simulink model "altitude_controller"  (R2019b)
settings: Solver=ode45  StartTime=0.0  StopTime=50  FixedStep=1e-3  RelTol=1e-5
InitFcn:
  | % load parameters of the default quadrotor
  | disp('Quadrotor parameters loaded by InitFcn')
  | mdl_quadrotor
undefined symbols (not defined in the file or in its folder): A, B, C, D, pwm, quad
libraries: realtime_pacer_lib x2, simulink x1
settings Model: Creator=corkep  LastModifiedBy=lab
settings DataIOCC: LimitDataPoints=on  SaveFormat=Array  SignalLoggingSaveFormat=ModelDataLogs  ReturnWorkspaceOutputs=off
settings OptimizationCC: BlockReduction=off  BooleanDataType=off  LifeSpan=inf
settings DebuggingCC: SaveWithParameterizedLinksMsg=none  UnderspecifiedInitializationDetection=Classic  MergeDetectMultiDrivingBlocksExec=none  SignalResolutionControl=TryResolveAllWithWarning  MultiTaskDSMMsg=warning  MultiTaskCondExecSysMsg=none  AllowSymbolicDim=off  StateNameClashWarn=warning  SFUnexpectedBacktrackingDiag=warning  SFNoUnconditionalDefaultTransitionDiag=warning  SFExecutionAtInitializationDiag=none  ArithmeticOperatorsInVariantConditions=warning
settings HardwareCC: ProdBitPerPointer=32  ProdBitPerSizeT=32  ProdBitPerPtrDiffT=32  ProdLargestAtomicFloat=None  ProdIntDivRoundTo=Undefined  ProdEndianess=Unspecified  ProdWordSize=32  ProdHWDeviceType=32-bit Generic  TargetUnknown=on
settings ModelReferenceCC: PropagateSignalLabelsOutOfModel=off
settings SFSimCC: SimUseLocalCustomCode=off  CustomCodeUndefinedFunction=UseInterfaceOnly
settings RTWCC: RTWUseLocalCustomCode=off
settings CodeAppCC: StateflowObjectComments=on
settings GRTTargetCC: TargetLangStandard=C89/C90 (ANSI)  GeneratePreprocessorConditionals=Disable all
settings ConfigComp: CovMetricSettings=dw  CovHtmlReporting=on  CovSaveCumulativeToWorkspaceVar=on  CovSaveSingleToWorkspaceVar=on  CovExternalEMLEnable=off

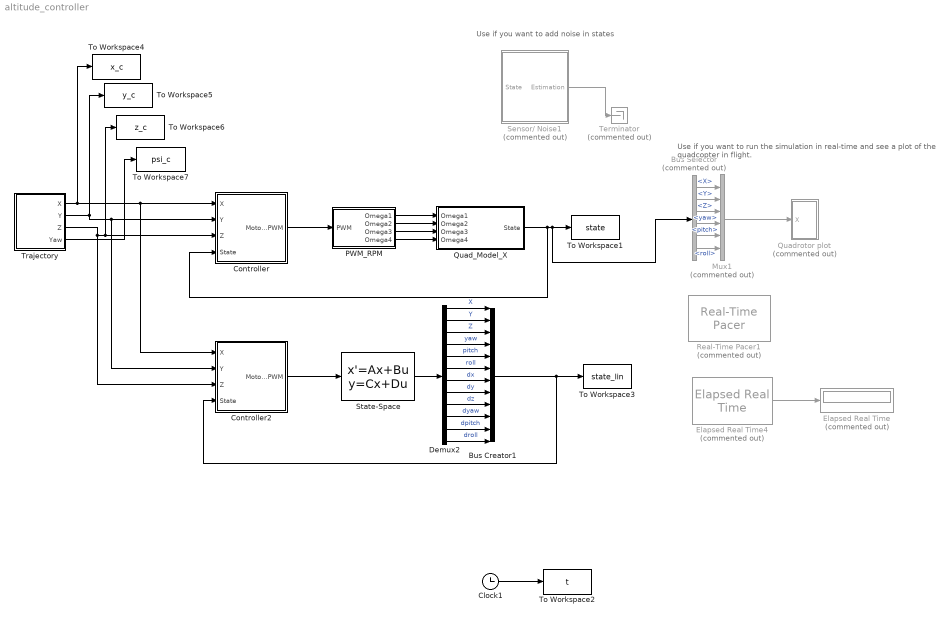
== system altitude_controller ==
  note: Use if you want to run the simulation in real-time and see
      | a plot of the quadcopter in flight.
  note: Use if you want to add noise in states
  Bus Creator1 : BusCreator  Inputs=12
  Bus Selector : BusSelector  Commented=on  OutputSignals=X,Y,Z,yaw,pitch,roll
  Clock1 : Clock
  Controller : Subsystem  TreatAsAtomicUnit=on
  Controller2 : Subsystem  TreatAsAtomicUnit=on
  Demux2 : Demux  Outputs=12
  Elapsed Real Time : Display  Commented=on
      settings: Decimation=2
  Elapsed Real Time4 : realtime_pacer_lib/Elapsed Real Time  Commented=on
  Mux1 : Mux  Commented=on  Inputs=6
  PWM_RPM : Subsystem
  Quad_Model_X : Subsystem
  Quadrotor plot : Subsystem  Commented=on  AncestorBlock=roblocks/Robot Graphics/Quadrotor plot  mask{quad=quad, xydim=2, zdim=2.3}
      mask prompts: quad "Model"; xydim "xy-axes dimension"; zdim "z-axis dimension"
      mask help: Animate quadrotor.
      mask Help:
      | This block graphically displays a quadrotor (flying robot).
      | 
      | A new figure is created and A graphical model of a quadrotor is animated
      | to a pose specified by the state vector input to the block.
      | 
      | The state vector is [x y z roll pitch yaw] in world coordinates and the
      | angles are in radians.
      | 
      | Notes:
      | - The dimensions of the vehicle workspace are set by parameters
  Real-Time Pacer1 : realtime_pacer_lib/Real-Time Pacer  Commented=on  simTimePerRealTime=1
  Sensor/ Noise1 : Subsystem  Commented=on
  State-Space : StateSpace  A=A  B=B  C=C  D=D  InitialCondition=[0 0 0 0 0 0 0 0 0 0 0 0]'
  Terminator : Terminator  Commented=on
  To Workspace1 : ToWorkspace  VariableName=state  SampleTime=-1
  To Workspace2 : ToWorkspace  VariableName=t  SampleTime=-1
  To Workspace3 : ToWorkspace  VariableName=state_lin  SampleTime=-1
  To Workspace4 : ToWorkspace  VariableName=x_c  SampleTime=-1
  To Workspace5 : ToWorkspace  VariableName=y_c  SampleTime=-1
  To Workspace6 : ToWorkspace  VariableName=z_c  SampleTime=-1
  To Workspace7 : ToWorkspace  VariableName=psi_c  SampleTime=-1
  Trajectory : Subsystem
  wires:
  Clock1/1 -> To Workspace2/1
  Trajectory/3(Z) -> Controller2/3(Z), To Workspace6/1, Controller/3(Z)
  Trajectory/4(Yaw) -> To Workspace7/1
  Controller2/1(Motors_PWM) -> State-Space/1
  Demux2/1 -> Bus Creator1/1  "X"
  Demux2/2 -> Bus Creator1/2  "Y"
  Demux2/3 -> Bus Creator1/3  "Z"
  Demux2/4 -> Bus Creator1/4  "yaw"
  Demux2/5 -> Bus Creator1/5  "pitch"
  Demux2/6 -> Bus Creator1/6  "roll"
  Demux2/7 -> Bus Creator1/7  "dx"
  Demux2/8 -> Bus Creator1/8  "dy"
  Demux2/9 -> Bus Creator1/9  "dz"
  Demux2/10 -> Bus Creator1/10  "dyaw"
  Demux2/11 -> Bus Creator1/11  "dpitch"
  Demux2/12 -> Bus Creator1/12  "droll"
  State-Space/1 -> Demux2/1
  Controller/1(Motors_PWM) -> PWM_RPM/1(PWM)
  Trajectory/2(Y) -> To Workspace5/1, Controller2/2(Y), Controller/2(Y)
  Trajectory/1(X) -> To Workspace4/1, Controller2/1(X), Controller/1(X)
  PWM_RPM/1(Omega1) -> Quad_Model_X/1(Omega1)
  PWM_RPM/2(Omega2) -> Quad_Model_X/2(Omega2)
  PWM_RPM/3(Omega3) -> Quad_Model_X/3(Omega3)
  PWM_RPM/4(Omega4) -> Quad_Model_X/4(Omega4)
  Sensor/ Noise1/1(Estimation) -> Terminator/1
  Bus Creator1/1 -> Controller2/4(State), To Workspace3/1
  Mux1/1 -> Quadrotor plot/1(X)
  Bus Selector/6 -> Mux1/6  "<roll>"
  Bus Selector/5 -> Mux1/5  "<pitch>"
  Bus Selector/4 -> Mux1/4  "<yaw>"
  Bus Selector/3 -> Mux1/3  "<Z>"
  Bus Selector/2 -> Mux1/2  "<Y>"
  Bus Selector/1 -> Mux1/1  "<X>"
  Elapsed Real Time4/1 -> Elapsed Real Time/1
  Quad_Model_X/1(State) -> Controller/4(State), Bus Selector/1, To Workspace1/1

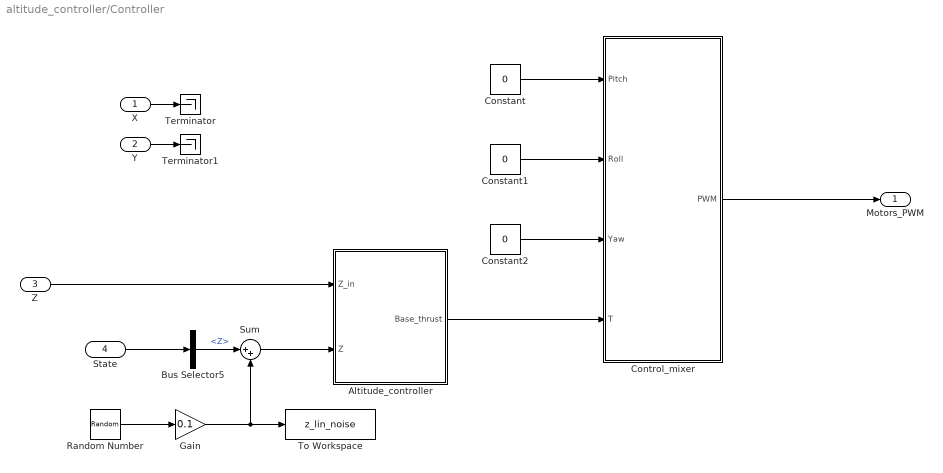
== system altitude_controller/Controller ==
  X : Inport
  Y : Inport  Port=2
  Z : Inport  Port=3
  State : Inport  Port=4
  Altitude_controller : Subsystem
  Bus Selector5 : BusSelector  OutputSignals=Z
  Constant : Constant  Value=0
  Constant1 : Constant  Value=0
  Constant2 : Constant  Value=0
  Control_mixer : Subsystem
  Gain : Gain  Gain=0.1
  Random Number : RandomNumber  SampleTime=0.01
  Sum : Sum  Inputs=|++
  Terminator : Terminator
  Terminator1 : Terminator
  To Workspace : ToWorkspace  VariableName=z_lin_noise  SaveFormat=Timeseries  SampleTime=-1
  Motors_PWM : Outport
  wires:
  Control_mixer/1(PWM) -> Motors_PWM/1
  Altitude_controller/1(Base_thrust) -> Control_mixer/4(T)
  Z/1 -> Altitude_controller/1(Z_in)
  Sum/1 -> Altitude_controller/2(Z)
  State/1 -> Bus Selector5/1
  Constant/1 -> Control_mixer/1(Pitch)
  Constant1/1 -> Control_mixer/2("Roll\t")
  Constant2/1 -> Control_mixer/3(Yaw)
  X/1 -> Terminator/1
  Y/1 -> Terminator1/1
  Bus Selector5/1 -> Sum/1  "<Z>"
  Random Number/1 -> Gain/1
  Gain/1 -> Sum/2, To Workspace/1

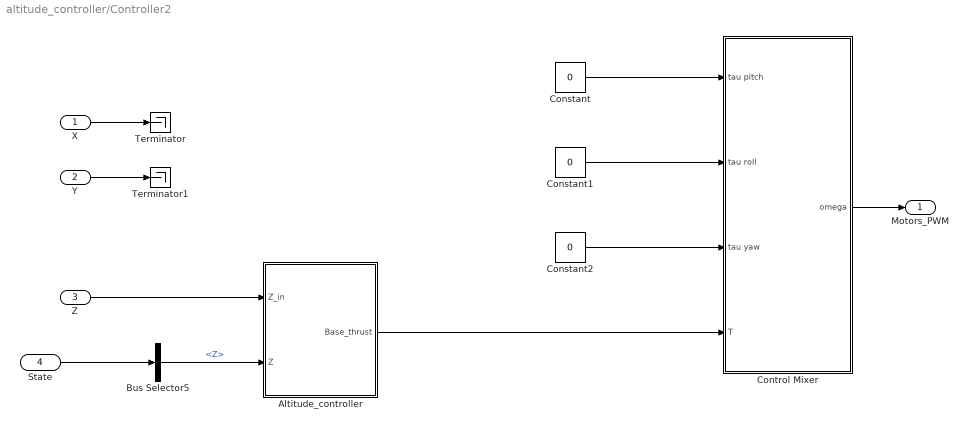
== system altitude_controller/Controller2 ==
  X : Inport
  Y : Inport  Port=2
  Z : Inport  Port=3
  State : Inport  Port=4
  Altitude_controller : Subsystem
  Bus Selector5 : BusSelector  OutputSignals=Z
  Constant : Constant  Value=0
  Constant1 : Constant  Value=0
  Constant2 : Constant  Value=0
  Control Mixer : Subsystem  AncestorBlock=roblocks/Dynamics/Control Mixer 4
      mask help: Quadrotor control mixer
      mask Help:
      | Determine rotor speeds based on desired torques and thrust.
      | 
      | <b>Inputs::</b>
      | 
      | tau pitch (1x1)  desired pitching torque [Nm]
      | tau roll (1x1)   desired rolling torque [Nm]
      | tau yaw (1x1)    desired yawing torque [Nm]
      | T (1x1)          desired thrust [N]
      | 
      | <b>Outputs::</b>
      | 
      | w1 (1x1) angular velocity of rotor 1 [rad]
      | w2 (1x1) angular velocity of rotor 2 [rad]
      | w3 (1x1) angular velocity of rotor 3 [rad]
      | w4 (1x1) angular velocity of rotor 4 [rad]
      | 
      | <b>Notes::</b>
      | 
      | - Assumes the rotor labelling convention of RVC Fig 4.16.
      | - The quadrotor is underactuated and has only 4 inputs.
  Terminator : Terminator
  Terminator1 : Terminator
  Motors_PWM : Outport
  wires:
  Constant2/1 -> Control Mixer/3(tau yaw)
  State/1 -> Bus Selector5/1
  Bus Selector5/1 -> Altitude_controller/2(Z)  "<Z>"
  Z/1 -> Altitude_controller/1(Z_in)
  Altitude_controller/1(Base_thrust) -> Control Mixer/4(T)
  Constant1/1 -> Control Mixer/2(tau roll)
  Constant/1 -> Control Mixer/1(tau pitch)
  Control Mixer/1(omega) -> Motors_PWM/1
  X/1 -> Terminator/1
  Y/1 -> Terminator1/1

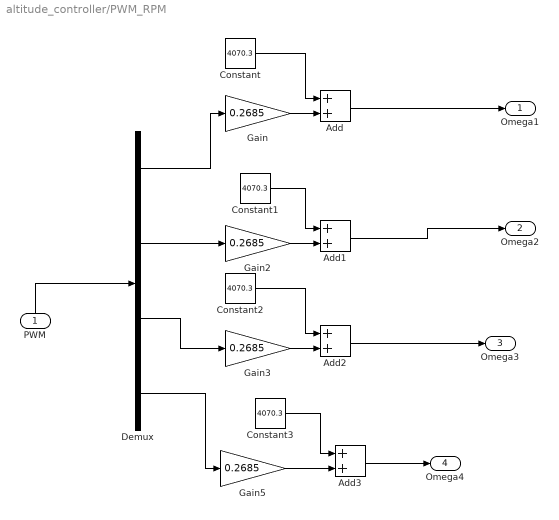
== system altitude_controller/PWM_RPM ==
  PWM : Inport
  Add{,1..3} (4 alike) : Sum
  Constant{,1..3} (4 alike) : Constant  Value=4070.3
  Demux : Demux
  Gain{,2..3,5} (4 alike) : Gain  Gain=0.2685
  Omega1 : Outport
  Omega2 : Outport  Port=2
  Omega3 : Outport  Port=3
  Omega4 : Outport  Port=4
  wires:
  Gain/1 -> Add/2
  Demux/1 -> Gain/1
  Demux/4 -> Gain5/1
  Gain5/1 -> Add3/2
  Constant3/1 -> Add3/1
  Add3/1 -> Omega4/1
  Constant1/1 -> Add1/1
  Gain2/1 -> Add1/2
  Demux/2 -> Gain2/1
  Add1/1 -> Omega2/1
  PWM/1 -> Demux/1
  Add/1 -> Omega1/1
  Add2/1 -> Omega3/1
  Demux/3 -> Gain3/1
  Constant2/1 -> Add2/1
  Gain3/1 -> Add2/2
  Constant/1 -> Add/1

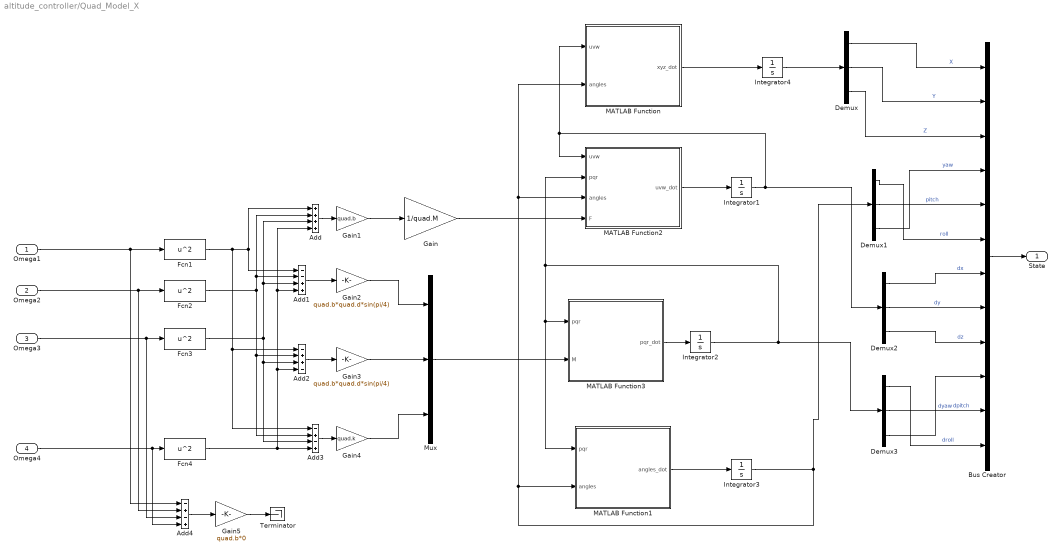
== system altitude_controller/Quad_Model_X ==
  Omega1 : Inport
  Omega2 : Inport  Port=2
  Omega3 : Inport  Port=3
  Omega4 : Inport  Port=4
  Add : Sum  Inputs=++++
  Add1 : Sum  Inputs=--++
  Add2 : Sum  Inputs=-++-
  Add3 : Sum  Inputs=-+-+
  Add4 : Sum  Inputs=-+-+
  Bus Creator : BusCreator  Inputs=12
  Demux{,1..3} (4 alike) : Demux  Outputs=3
  Fcn{1..4} (4 alike) : Fcn  Expr=u^2
  Gain : Gain  Gain=1/quad.M
  Gain1 : Gain  Gain=quad.b
  Gain2 : Gain  Gain=quad.b*quad.d*sin(pi/4)
  Gain3 : Gain  Gain=quad.b*quad.d*sin(pi/4)
  Gain4 : Gain  Gain=quad.k
  Gain5 : Gain  Gain=quad.b*0
  Integrator1 : Integrator
  Integrator2 : Integrator
  Integrator3 : Integrator
  Integrator4 : Integrator  InitialCondition=[0;0;0]
  MATLAB Function : MATLAB Function  TreatAsAtomicUnit=on
  MATLAB Function1 : MATLAB Function  TreatAsAtomicUnit=on
  MATLAB Function2 : MATLAB Function  TreatAsAtomicUnit=on
  MATLAB Function3 : MATLAB Function  TreatAsAtomicUnit=on
  Mux : Mux  Inputs=3
  Terminator : Terminator
  State : Outport
  wires:
  Gain1/1 -> Gain/1
  Fcn4/1 -> Add/4, Add1/4, Add2/4, Add3/4
  Fcn3/1 -> Add1/3, Add/3, Add2/3, Add3/3
  Fcn2/1 -> Add2/2, Add3/2, Add1/2, Add/2
  Fcn1/1 -> Add/1, Add1/1, Add2/1, Add3/1
  Bus Creator/1 -> State/1
  Add1/1 -> Gain2/1
  Add/1 -> Gain1/1
  Omega2/1 -> Add4/2, Fcn2/1
  Omega1/1 -> Fcn1/1, Add4/1
  Add2/1 -> Gain3/1
  Gain2/1 -> Mux/1
  Gain4/1 -> Mux/3
  Omega3/1 -> Add4/3, Fcn3/1
  Omega4/1 -> Fcn4/1, Add4/4
  Add4/1 -> Gain5/1
  Add3/1 -> Gain4/1
  Gain3/1 -> Mux/2
  Gain/1 -> MATLAB Function2/4(F)
  Mux/1 -> MATLAB Function3/2(M)
  MATLAB Function/1(xyz_dot) -> Integrator4/1
  MATLAB Function2/1(uvw_dot) -> Integrator1/1
  MATLAB Function3/1(pqr_dot) -> Integrator2/1
  MATLAB Function1/1(angles_dot) -> Integrator3/1
  Integrator3/1 -> Demux1/1, MATLAB Function/2(angles), MATLAB Function2/3(angles), MATLAB Function1/2(angles)
  Integrator1/1 -> Demux2/1, MATLAB Function/1(uvw), MATLAB Function2/1(uvw)
  Integrator2/1 -> Demux3/1, MATLAB Function2/2(pqr), MATLAB Function1/1(pqr), MATLAB Function3/1(pqr)
  Integrator4/1 -> Demux/1
  Demux/1 -> Bus Creator/1  "X"
  Demux/2 -> Bus Creator/2  "Y"
  Demux/3 -> Bus Creator/3  "Z"
  Demux1/3 -> Bus Creator/4  "yaw"
  Demux1/1 -> Bus Creator/6  "roll"
  Demux2/1 -> Bus Creator/7  "dx"
  Demux2/2 -> Bus Creator/8  "dy"
  Demux2/3 -> Bus Creator/9  "dz"
  Demux3/3 -> Bus Creator/10  "dyaw"
  Demux3/2 -> Bus Creator/11  "dpitch"
  Demux3/1 -> Bus Creator/12  "droll"
  Gain5/1 -> Terminator/1
  Demux1/2 -> Bus Creator/5  "pitch"

== system altitude_controller/Quadrotor plot ==
  X : Inport
  Plotter : S-Function  FunctionName=quadrotor_plot  Parameters=[xydim, zdim], 1, 1,quad  SFunctionDeploymentMode=off  EnableBusSupport=off
  wires:
  X/1 -> Plotter/1

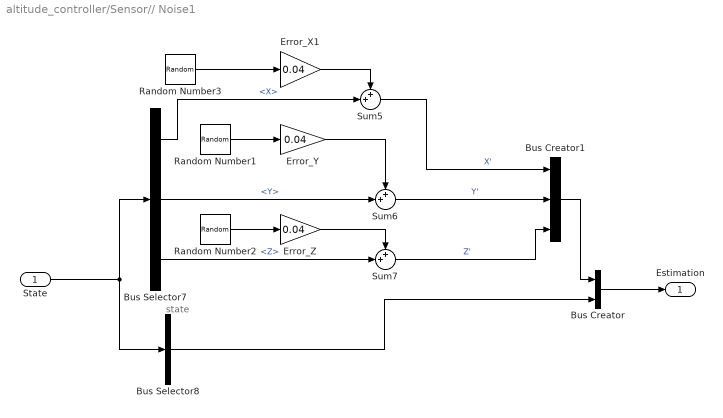
== system altitude_controller/Sensor// Noise1 ==
  note: state
  State : Inport
  Bus Creator : BusCreator  Inputs=2
  Bus Creator1 : BusCreator  Inputs=3
  Bus Selector7 : BusSelector  OutputSignals=X,Y,Z
  Bus Selector8 : BusSelector  OutputSignals=yaw,pitch,roll,dx,dy,dz,dyaw,dpitch,droll  OutputAsBus=on
  Error_X1 : Gain  Gain=0.04
  Error_Y : Gain  Gain=0.04
  Error_Z : Gain  Gain=0.04
  Random Number1 : RandomNumber  SampleTime=0.1
  Random Number2 : RandomNumber  SampleTime=0.1
  Random Number3 : RandomNumber  SampleTime=0.1
  Sum5 : Sum  Inputs=++|
  Sum6 : Sum  Inputs=++|
  Sum7 : Sum  Inputs=++|
  Estimation : Outport
  wires:
  State/1 -> Bus Selector8/1, Bus Selector7/1
  Error_X1/1 -> Sum5/1
  Bus Selector8/1 -> Bus Creator/2
  Random Number3/1 -> Error_X1/1
  Bus Creator/1 -> Estimation/1
  Bus Selector7/1 -> Sum5/2  "<X>"
  Bus Selector7/2 -> Sum6/2  "<Y>"
  Bus Selector7/3 -> Sum7/2  "<Z>"
  Sum5/1 -> Bus Creator1/1  "X'"
  Sum6/1 -> Bus Creator1/2  "Y'"
  Sum7/1 -> Bus Creator1/3  "Z'"
  Bus Creator1/1 -> Bus Creator/1
  Random Number1/1 -> Error_Y/1
  Error_Y/1 -> Sum6/1
  Random Number2/1 -> Error_Z/1
  Error_Z/1 -> Sum7/1

== system altitude_controller/Trajectory ==
  Constant3 : Constant
  Ramp2 : simulink/Sources/Ramp  slope=60  start=0  InitialOutput=0
  x* : Sin  Amplitude=0.8  Frequency=2*pi*0.085  Phase=0-0.1  SampleTime=0
  y*1 : Sin  Amplitude=0.8  Frequency=2*pi*0.085  Phase=pi/2-0.1  SampleTime=0
  X : Outport
  Y : Outport  Port=2
  Z : Outport  Port=3
  Yaw : Outport  Port=4
  wires:
  Ramp2/1 -> Yaw/1
  y*1/1 -> Y/1
  x*/1 -> X/1
  Constant3/1 -> Z/1

== system altitude_controller/Controller/Altitude_controller ==
  Z_in : Inport
  Z : Inport  Port=2
  "Min_thrust " : Constant  Value=pwm  SampleTime=0
  PID_Altitude : Subsystem
  Saturation : Saturate  UpperLimit=60000  LowerLimit=-20000
  Saturation1 : Saturate  UpperLimit=15000  LowerLimit=-20000
  Sum3 : Sum  Inputs=|++
  Base_thrust : Outport
  wires:
  Saturation/1 -> Base_thrust/1
  "Min_thrust "/1 -> Sum3/2
  Sum3/1 -> Saturation/1
  Z/1 -> PID_Altitude/2(Measured)
  Z_in/1 -> PID_Altitude/1(Setpoint)
  Saturation1/1 -> Sum3/1
  PID_Altitude/1(Adjust) -> Saturation1/1

== system altitude_controller/Controller/Control_mixer ==
  Pitch : Inport
  "Roll\t" : Inport  Port=2
  Yaw : Inport  Port=3
  T : Inport  Port=4
  Configuration_+ : Subsystem
  Configuration_X1 : Subsystem
  Mode_Selector : Constant  Value=2
  Multiport Switch : MultiPortSwitch  Inputs=2
  Mux : Mux
  Mux1 : Mux
  PWM : Outport
  wires:
  Pitch/1 -> Configuration_X1/1(Pitch), Configuration_+/1(Pitch)
  Configuration_X1/3(W3) -> Mux1/3
  Mux1/1 -> Multiport Switch/3
  Mux/1 -> Multiport Switch/2
  Configuration_X1/4(W4) -> Mux1/4
  T/1 -> Configuration_X1/4(Tau), Configuration_+/4(Tau)
  Multiport Switch/1 -> PWM/1
  Yaw/1 -> Configuration_X1/3(Yaw), Configuration_+/3(Yaw)
  "Roll\t"/1 -> Configuration_X1/2(Roll), Configuration_+/2(Roll)
  Mode_Selector/1 -> Multiport Switch/1
  Configuration_+/2(W2) -> Mux/2
  Configuration_+/1(W1) -> Mux/1
  Configuration_X1/2(W2) -> Mux1/2
  Configuration_X1/1(W1) -> Mux1/1
  Configuration_+/3(W3) -> Mux/3
  Configuration_+/4(W4) -> Mux/4

== system altitude_controller/Controller2/Altitude_controller ==
  Z_in : Inport
  Z : Inport  Port=2
  "Min_thrust " : Constant  Value=0  SampleTime=0
  PID_Altitude : Subsystem
  Saturation : Saturate  UpperLimit=60000  LowerLimit=-20000
  Saturation1 : Saturate  UpperLimit=15000  LowerLimit=-20000
  Sum3 : Sum  Inputs=|++
  Base_thrust : Outport
  wires:
  PID_Altitude/1(Adjust) -> Sum3/1
  Saturation1/1 -> ?
  Z_in/1 -> PID_Altitude/1(Setpoint)
  Z/1 -> PID_Altitude/2(Measured)
  Sum3/1 -> Base_thrust/1
  "Min_thrust "/1 -> Sum3/2
  Saturation/1 -> ?

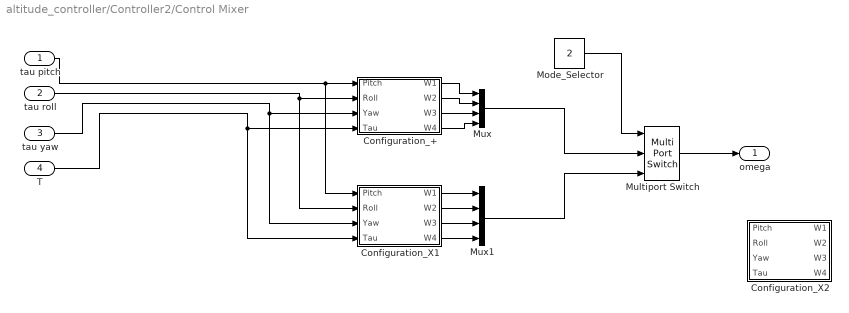
== system altitude_controller/Controller2/Control Mixer ==
  tau pitch : Inport
  tau roll : Inport  Port=2
  tau yaw : Inport  Port=3
  T : Inport  Port=4
  Configuration_+ : Subsystem
  Configuration_X1 : Subsystem
  Configuration_X2 : Subsystem
  Mode_Selector : Constant  Value=2
  Multiport Switch : MultiPortSwitch  Inputs=2
  Mux : Mux
  Mux1 : Mux
  omega : Outport
  wires:
  Mux/1 -> Multiport Switch/2
  Multiport Switch/1 -> omega/1
  Mode_Selector/1 -> Multiport Switch/1
  T/1 -> Configuration_+/4(Tau), Configuration_X1/4(Tau)
  tau yaw/1 -> Configuration_+/3(Yaw), Configuration_X1/3(Yaw)
  tau roll/1 -> Configuration_+/2(Roll), Configuration_X1/2(Roll)
  tau pitch/1 -> Configuration_+/1(Pitch), Configuration_X1/1(Pitch)
  Mux1/1 -> Multiport Switch/3
  Configuration_X1/4(W4) -> Mux1/4
  Configuration_X1/3(W3) -> Mux1/3
  Configuration_X1/2(W2) -> Mux1/2
  Configuration_X1/1(W1) -> Mux1/1
  Configuration_+/4(W4) -> Mux/4
  Configuration_+/3(W3) -> Mux/3
  Configuration_+/2(W2) -> Mux/2
  Configuration_+/1(W1) -> Mux/1

== system altitude_controller/Controller/Altitude_controller/PID_Altitude ==
  Setpoint : Inport
  Measured : Inport  Port=2
  Derivative : Derivative
  Integrator Limited : Integrator  LimitOutput=on  UpperSaturationLimit=1000  LowerSaturationLimit=-1000
  Kd : Gain  Gain=9000  OutMin=[-200]  OutMax=[200]
  Ki : Gain  Gain=3500  OutMin=[-200]  OutMax=[200]
  Kp : Gain  Gain=11000  OutMin=[-200]  OutMax=[200]
  Sum5 : Sum  Inputs=+++
  Sum6 : Sum  Inputs=+-|
  Adjust : Outport
  wires:
  Derivative/1 -> Kd/1
  Integrator Limited/1 -> Ki/1
  Sum6/1 -> Kp/1, Integrator Limited/1, Derivative/1  "pid_error"
  Kd/1 -> Sum5/3
  Kp/1 -> Sum5/1
  Ki/1 -> Sum5/2
  Setpoint/1 -> Sum6/1  "pid_desired"
  Measured/1 -> Sum6/2  "measured"
  Sum5/1 -> Adjust/1

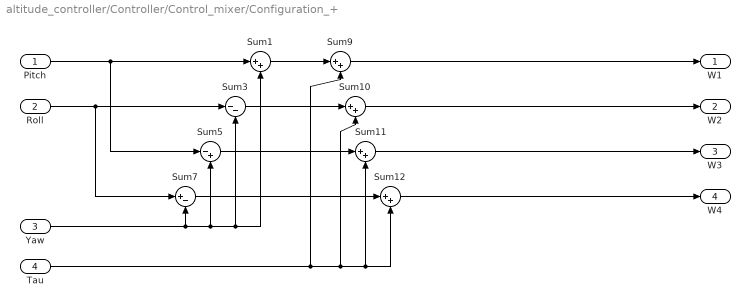
== system altitude_controller/Controller/Control_mixer/Configuration_+ ==
  Pitch : Inport
  Roll : Inport  Port=2
  Yaw : Inport  Port=3
  Tau : Inport  Port=4
  Sum{1,9..12} (5 alike) : Sum  Inputs=|++  SaturateOnIntegerOverflow=on  InputSameDT=on  OutDataTypeStr=Inherit: Same as first input
  Sum3 : Sum  Inputs=|--  SaturateOnIntegerOverflow=on  InputSameDT=on  OutDataTypeStr=Inherit: Same as first input
  Sum5 : Sum  Inputs=|-+  SaturateOnIntegerOverflow=on  InputSameDT=on  OutDataTypeStr=Inherit: Same as first input
  Sum7 : Sum  Inputs=|+-  SaturateOnIntegerOverflow=on  InputSameDT=on  OutDataTypeStr=Inherit: Same as first input
  W1 : Outport
  W2 : Outport  Port=2
  W3 : Outport  Port=3
  W4 : Outport  Port=4
  wires:
  Sum5/1 -> Sum11/1
  Yaw/1 -> Sum7/2, Sum5/2, Sum3/2, Sum1/2
  Tau/1 -> Sum11/2, Sum12/2, Sum10/2, Sum9/2
  Sum9/1 -> W1/1
  Pitch/1 -> Sum1/1, Sum5/1
  Roll/1 -> Sum3/1, Sum7/1
  Sum11/1 -> W3/1
  Sum12/1 -> W4/1
  Sum7/1 -> Sum12/1
  Sum10/1 -> W2/1
  Sum1/1 -> Sum9/1
  Sum3/1 -> Sum10/1

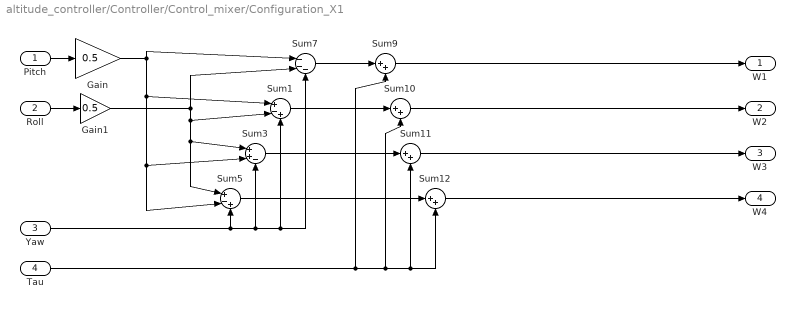
== system altitude_controller/Controller/Control_mixer/Configuration_X1 ==
  Pitch : Inport
  Roll : Inport  Port=2
  Yaw : Inport  Port=3
  Tau : Inport  Port=4
  Gain : Gain  Gain=0.5
  Gain1 : Gain  Gain=0.5
  Sum1 : Sum  Inputs=|+-+  SaturateOnIntegerOverflow=on  InputSameDT=on  OutDataTypeStr=Inherit: Same as first input
  Sum{9..12} (4 alike) : Sum  Inputs=|++  SaturateOnIntegerOverflow=on  InputSameDT=on  OutDataTypeStr=Inherit: Same as first input
  Sum3 : Sum  Inputs=|++-  SaturateOnIntegerOverflow=on  InputSameDT=on  OutDataTypeStr=Inherit: Same as first input
  Sum5 : Sum  Inputs=|+-+  SaturateOnIntegerOverflow=on  InputSameDT=on  OutDataTypeStr=Inherit: Same as first input
  Sum7 : Sum  Inputs=|---  SaturateOnIntegerOverflow=on  InputSameDT=on  OutDataTypeStr=Inherit: Same as first input
  W1 : Outport
  W2 : Outport  Port=2
  W3 : Outport  Port=3
  W4 : Outport  Port=4
  wires:
  Sum3/1 -> Sum11/1
  Yaw/1 -> Sum5/3, Sum3/3, Sum7/3, Sum1/3
  Tau/1 -> Sum11/2, Sum12/2, Sum10/2, Sum9/2
  Sum5/1 -> Sum12/1
  Sum7/1 -> Sum9/1
  Sum1/1 -> Sum10/1
  Roll/1 -> Gain1/1
  Pitch/1 -> Gain/1
  Gain/1 -> Sum7/1, Sum1/1, Sum5/2, Sum3/2
  Gain1/1 -> Sum7/2, Sum1/2, Sum5/1, Sum3/1
  Sum9/1 -> W1/1
  Sum10/1 -> W2/1
  Sum11/1 -> W3/1
  Sum12/1 -> W4/1

== system altitude_controller/Controller2/Altitude_controller/PID_Altitude ==
  Setpoint : Inport
  Measured : Inport  Port=2
  Derivative : Derivative
  Integrator Limited : Integrator  LimitOutput=on  UpperSaturationLimit=1000  LowerSaturationLimit=-1000
  Kd : Gain  Gain=9000  OutMin=[-200]  OutMax=[200]
  Ki : Gain  Gain=3500  OutMin=[-200]  OutMax=[200]
  Kp : Gain  Gain=11000  OutMin=[-200]  OutMax=[200]
  Sum5 : Sum  Inputs=+++
  Sum6 : Sum  Inputs=+-|
  Adjust : Outport
  wires:
  Sum5/1 -> Adjust/1
  Measured/1 -> Sum6/2  "measured"
  Setpoint/1 -> Sum6/1  "pid_desired"
  Ki/1 -> Sum5/2
  Kp/1 -> Sum5/1
  Kd/1 -> Sum5/3
  Sum6/1 -> Derivative/1, Integrator Limited/1, Kp/1  "pid_error"
  Integrator Limited/1 -> Ki/1
  Derivative/1 -> Kd/1

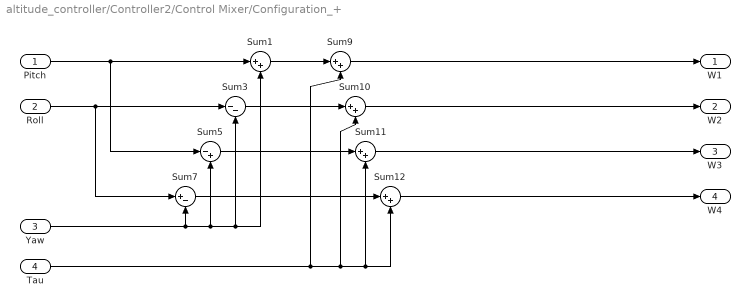
== system altitude_controller/Controller2/Control Mixer/Configuration_+ ==
  Pitch : Inport
  Roll : Inport  Port=2
  Yaw : Inport  Port=3
  Tau : Inport  Port=4
  Sum{1,9..12} (5 alike) : Sum  Inputs=|++  SaturateOnIntegerOverflow=on  InputSameDT=on  OutDataTypeStr=Inherit: Same as first input
  Sum3 : Sum  Inputs=|--  SaturateOnIntegerOverflow=on  InputSameDT=on  OutDataTypeStr=Inherit: Same as first input
  Sum5 : Sum  Inputs=|-+  SaturateOnIntegerOverflow=on  InputSameDT=on  OutDataTypeStr=Inherit: Same as first input
  Sum7 : Sum  Inputs=|+-  SaturateOnIntegerOverflow=on  InputSameDT=on  OutDataTypeStr=Inherit: Same as first input
  W1 : Outport
  W2 : Outport  Port=2
  W3 : Outport  Port=3
  W4 : Outport  Port=4
  wires:
  Sum3/1 -> Sum10/1
  Sum1/1 -> Sum9/1
  Sum10/1 -> W2/1
  Sum7/1 -> Sum12/1
  Sum12/1 -> W4/1
  Sum11/1 -> W3/1
  Roll/1 -> Sum7/1, Sum3/1
  Pitch/1 -> Sum5/1, Sum1/1
  Sum9/1 -> W1/1
  Tau/1 -> Sum9/2, Sum10/2, Sum12/2, Sum11/2
  Yaw/1 -> Sum1/2, Sum3/2, Sum5/2, Sum7/2
  Sum5/1 -> Sum11/1

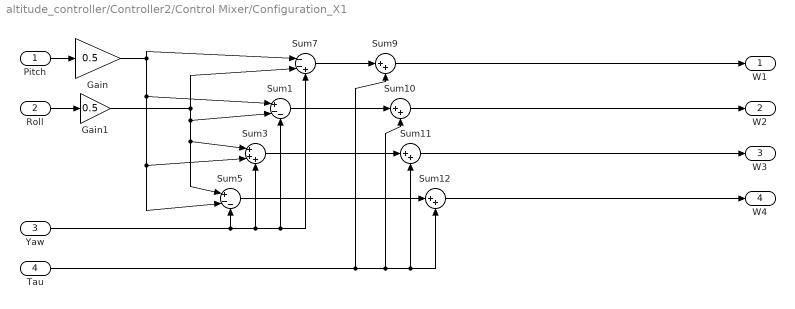
== system altitude_controller/Controller2/Control Mixer/Configuration_X1 ==
  Pitch : Inport
  Roll : Inport  Port=2
  Yaw : Inport  Port=3
  Tau : Inport  Port=4
  Gain : Gain  Gain=0.5
  Gain1 : Gain  Gain=0.5
  Sum1 : Sum  Inputs=|+--  SaturateOnIntegerOverflow=on  InputSameDT=on  OutDataTypeStr=Inherit: Same as first input
  Sum{9..12} (4 alike) : Sum  Inputs=|++  SaturateOnIntegerOverflow=on  InputSameDT=on  OutDataTypeStr=Inherit: Same as first input
  Sum3 : Sum  Inputs=|+++  SaturateOnIntegerOverflow=on  InputSameDT=on  OutDataTypeStr=Inherit: Same as first input
  Sum5 : Sum  Inputs=|+--  SaturateOnIntegerOverflow=on  InputSameDT=on  OutDataTypeStr=Inherit: Same as first input
  Sum7 : Sum  Inputs=|--+  SaturateOnIntegerOverflow=on  InputSameDT=on  OutDataTypeStr=Inherit: Same as first input
  W1 : Outport
  W2 : Outport  Port=2
  W3 : Outport  Port=3
  W4 : Outport  Port=4
  wires:
  Sum12/1 -> W4/1
  Sum11/1 -> W3/1
  Sum10/1 -> W2/1
  Sum9/1 -> W1/1
  Gain1/1 -> Sum3/1, Sum5/1, Sum1/2, Sum7/2
  Gain/1 -> Sum3/2, Sum5/2, Sum1/1, Sum7/1
  Pitch/1 -> Gain/1
  Roll/1 -> Gain1/1
  Sum1/1 -> Sum10/1
  Sum7/1 -> Sum9/1
  Sum5/1 -> Sum12/1
  Tau/1 -> Sum9/2, Sum10/2, Sum12/2, Sum11/2
  Yaw/1 -> Sum1/3, Sum7/3, Sum3/3, Sum5/3
  Sum3/1 -> Sum11/1

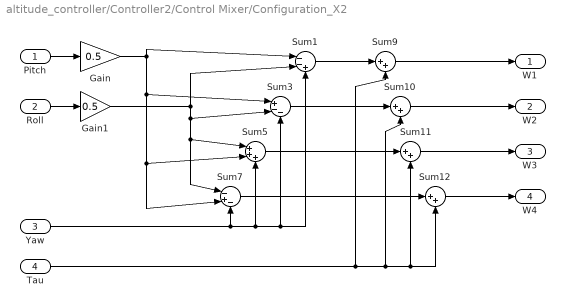
== system altitude_controller/Controller2/Control Mixer/Configuration_X2 ==
  Pitch : Inport
  Roll : Inport  Port=2
  Yaw : Inport  Port=3
  Tau : Inport  Port=4
  Gain : Gain  Gain=0.5
  Gain1 : Gain  Gain=0.5
  Sum1 : Sum  Inputs=|--+  SaturateOnIntegerOverflow=on  InputSameDT=on  OutDataTypeStr=Inherit: Same as first input
  Sum{9..12} (4 alike) : Sum  Inputs=|++  SaturateOnIntegerOverflow=on  InputSameDT=on  OutDataTypeStr=Inherit: Same as first input
  Sum3 : Sum  Inputs=|+--  SaturateOnIntegerOverflow=on  InputSameDT=on  OutDataTypeStr=Inherit: Same as first input
  Sum5 : Sum  Inputs=|+++  SaturateOnIntegerOverflow=on  InputSameDT=on  OutDataTypeStr=Inherit: Same as first input
  Sum7 : Sum  Inputs=|-+-  SaturateOnIntegerOverflow=on  InputSameDT=on  OutDataTypeStr=Inherit: Same as first input
  W1 : Outport
  W2 : Outport  Port=2
  W3 : Outport  Port=3
  W4 : Outport  Port=4
  wires:
  Sum5/1 -> Sum11/1
  Yaw/1 -> Sum7/3, Sum5/3, Sum1/3, Sum3/3
  Tau/1 -> Sum11/2, Sum12/2, Sum10/2, Sum9/2
  Sum7/1 -> Sum12/1
  Sum1/1 -> Sum9/1
  Sum3/1 -> Sum10/1
  Roll/1 -> Gain1/1
  Pitch/1 -> Gain/1
  Gain/1 -> Sum3/1, Sum7/2, Sum5/2, Sum1/1
  Gain1/1 -> Sum1/2, Sum3/2, Sum5/1, Sum7/1
  Sum9/1 -> W1/1
  Sum10/1 -> W2/1
  Sum11/1 -> W3/1
  Sum12/1 -> W4/1

== matlab function altitude_controller/Quad_Model_X/MATLAB Function ==
  data: uvw input; xyz_dot output; angles input
function xyz_dot  = Position(uvw,angles)
xyz_dot = zeros(3,1);
phi = angles(1); %*pi/180;
theta = angles(2); %*pi/180;
psi = angles(3); %*pi/180;
Tb_o = [cos(theta)*cos(psi)                                cos(theta)*sin(psi)                             -sin(theta)  ;   %BBF > Inertial rotation matrix
        sin(phi)*sin(theta)*cos(psi)-cos(phi)*sin(psi)    sin(phi)*sin(theta)*sin(psi)+cos(phi)*cos(psi)  sin(phi)*cos(theta) ;
        cos(phi)*sin(theta)*cos(psi)+sin(phi)*sin(psi)    cos(phi)*sin(theta)*sin(psi)-sin(phi)*cos(psi)   cos(phi)*cos(theta)];

xyz_dot = (Tb_o')*uvw;
end

== matlab function altitude_controller/Quad_Model_X/MATLAB Function1 ==
  data: pqr input; angles_dot output; angles input
function angles_dot  = Angle(pqr,angles)
angles_dot = zeros(3,1);
phi = angles(1); %*pi/180;
theta = angles(2); %*pi/180;

H = [1    sin(phi)*tan(theta)     cos(phi)*tan(theta)
     0       cos(phi)                 -sin(phi)   
     0       sin(phi)/cos(theta)    cos(phi)/cos(theta)];
angles_dot = H*pqr;
end

== matlab function altitude_controller/Quad_Model_X/MATLAB Function2 ==
  data: uvw input; uvw_dot output; pqr input; angles input; F input
function uvw_dot  = Forces(uvw,pqr,angles,F)
uvw_dot = zeros(3,1);
Force = [0;0;F];
g_o = [0;0;-9.81];
phi = angles(1); %*pi/180;
theta = angles(2); %*pi/180;
psi = angles(3); %*pi/180;
Tb_o = [cos(theta)*cos(psi)                                cos(theta)*sin(psi)                             -sin(theta)  ;   %BBF > Inertial rotation matrix
        sin(phi)*sin(theta)*cos(psi)-cos(phi)*sin(psi)    sin(phi)*sin(theta)*sin(psi)+cos(phi)*cos(psi)  sin(phi)*cos(theta) ;
        cos(phi)*sin(theta)*cos(psi)+sin(phi)*sin(psi)    cos(phi)*sin(theta)*sin(psi)-sin(phi)*cos(psi)   cos(phi)*cos(theta)];

uvw_dot = Force + Tb_o*g_o - cross(pqr,uvw);

end

== matlab function altitude_controller/Quad_Model_X/MATLAB Function3 ==
  data: pqr_dot output; pqr input; M input
function pqr_dot  = Moments(pqr,M)
pqr_dot = zeros(3,1);
Ixx =  1.395e-05;  %2.3951e-5; %1.39e-05; %2.51943e-5; % % %
Iyy = 1.436e-05; %2.3951e-5; %1.436e-05; % 2.54379e-5; % %         %
Izz =  2.173e-05;  %3.2347e-5; %2.173e-05 ; %4.51407e-5; % %         %;%0.160;
J = diag([Ixx Iyy Izz]);    %   I  Flyer rotational inertia matrix     3x3
pqr_dot = inv(J)*(M-cross(pqr,J*pqr));
end
